simulink model "Solar_Panel_Tracking_Model"  (R2024b)
settings: Solver=VariableStepAuto  StartTime=0.0  StopTime=100  RelTol=1e-3
values from neighbouring files (symbols this model uses):
  J = 8.6    [Solar_Panel_Tracking_System.m]
  Kd = 8.6    [Solar_Panel_Tracking_System.m]
  Kf = 0.5    [Solar_Panel_Tracking_System.m]
  Kg = 1    [Solar_Panel_Tracking_System.m]
  Ki = 180    [Solar_Panel_Tracking_System.m]
  Kp = 240    [Solar_Panel_Tracking_System.m]
  Kt = 2    [Solar_Panel_Tracking_System.m]
  L = 1    [Solar_Panel_Tracking_System.m]
  R = 1.2    [Solar_Panel_Tracking_System.m]
libraries: slpidlib x1
settings Model: Creator=alexpadrpm  LastModifiedBy=alexpadrpm

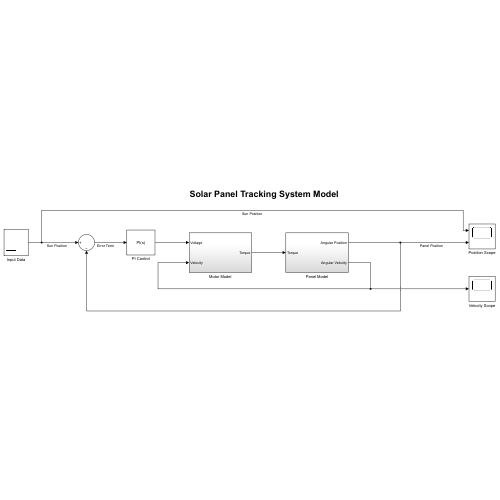
[thumbnail: Simulink's stored preview of the top-level diagram]
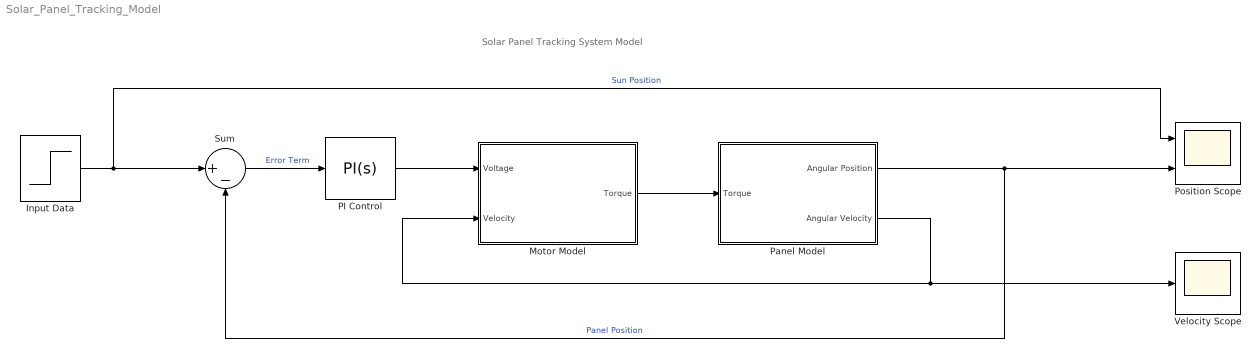
== system Solar_Panel_Tracking_Model ==
  note: Solar Panel Tracking System Model
  Input Data : Step  SampleTime=0
  Motor Model : Subsystem
  PI Control : slpidlib/PID Controller  Controller=PI  Form=Parallel  TimeDomain=Continuous-time  UseExternalTs=off  SampleTime=-1  IntegratorMethod=Forward Euler  FilterMethod=Forward Euler  ControllerParametersSource=internal  P=Kp  I=Ki  UseKiTs=off  D=0  UseExternalDerivativeSource=off  N=100  UseFilter=on  TunerSelectOption=Transfer Function Based (PID Tuner App)  InitialConditionSource=internal  InitialConditionForIntegrator=0  InitialConditionForFilter=0  DifferentiatorICPrevScaledInput=0  ExternalReset=none  TrackingMode=off  Kt=1  LimitOutput=off  SatLimitsSource=internal  UpperSaturationLimit=inf  LowerSaturationLimit=-inf  LinearizeAsGain=on  AntiWindupMode=none  Kb=1  LimitIntegrator=off  UpperIntegratorSaturationLimit=inf  LowerIntegratorSaturationLimit=-inf  POutMin=[]  POutMax=[]  IOutMin=[]  IOutMax=[]  DOutMin=[]  DOutMax=[]  NOutMin=[]  NOutMax=[]  SumOutMin=[]  SumOutMax=[]  SaturationOutMin=[]  SaturationOutMax=[]  PParamMin=[]  PParamMax=[]  IParamMin=[]  IParamMax=[]  DParamMin=[]  DParamMax=[]  NParamMin=[]  NParamMax=[]  KbParamMin=[]  KbParamMax=[]  KtParamMin=[]  KtParamMax=[]  KbOutMin=[]  KbOutMax=[]  KtOutMin=[]  KtOutMax=[]  IntegratorOutMin=[]  IntegratorOutMax=[]  FilterOutMin=[]  FilterOutMax=[]  SumI1OutMin=[]  SumI1OutMax=[]  SumI2OutMin=[]  SumI2OutMax=[]  SumI3OutMin=[]  SumI3OutMax=[]  SumI4OutMin=[]  SumI4OutMax=[]  SumDOutMin=[]  SumDOutMax=[]  DifferentiatorOutMin=[]  DifferentiatorOutMax=[]  FilterDiffOutCoefMin=[]  FilterDiffOutCoefMax=[]  ReciprocalOutMin=[]  ReciprocalOutMax=[]  SumDenOutMin=[]  SumDenOutMax=[]  SumNumOutMin=[]  SumNumOutMax=[]  DivideOutMin=[]  DivideOutMax=[]  UdiffTsProdOutMin=[]  UdiffTsProdOutMax=[]  NTsProdOutMin=[]  NTsProdOutMax=[]  UintegralTsProdOutMin=[]  UintegralTsProdOutMax=[]  UngainTsProdOutMin=[]  UngainTsProdOutMax=[]  ClampingZeroOutDataTypeStr=Inherit: Inherit via back propagation  ClampingZeroOutMin=[]  ClampingZeroOutMax=[]  FilterDenConstantOutDataTypeStr=Inherit: Inherit via back propagation  FilterDenConstantOutMin=[]  FilterDenConstantOutMax=[]  PCopyOutDataTypeStr=Inherit: Inherit via back propagation  PCopyOutMin=[]  PCopyOutMax=[]  NCopyOutDataTypeStr=Inherit: Inherit via back propagation  NCopyOutMin=[]  NCopyOutMax=[]  IntegratorContinuousStateAttributes=''  IntegratorStateMustResolveToSignalObject=off  IntegratorRTWStateStorageClass=Auto  FilterContinuousStateAttributes=''  FilterStateMustResolveToSignalObject=off  FilterRTWStateStorageClass=Auto  ParallelPVariant=InternalParameters  IdealPVariant=Disabled  IVariant=InternalParameters  DVariant=Disabled  IntegratorVariant=Continuous  SatVariant=Disabled  AWVariant=Passthrough  PCopyVariant=Disabled  TRVariant=Disabled  FdbkBlocksVariant=Forward  IdealPFdbkVariant=Disabled  SatFdbkVariant=Disabled  DerivativeFilterVariant=Disabled  NVariant=Disabled  NCopyVariant=Disabled_SignalSpec  FilterICVariant=Disabled  IntegratorICVariant=InternalICs  ExternalResetVariant=Disabled  TRSumVariant=Passthrough  SumFdbkVariant=Disabled  SumVariant=Sum_PI  TsampFilterVariant=InternalTs  TsampNgainVariant=Passthrough  TsampIntegralVariant=Disabled_SignalSpec  ExternalSaturationOutDataTypeStr=Inherit: Same as second input  DerivativeSourceVariant=Disabled  PreIntVariant=InternalPreInt
  Panel Model : Subsystem
  Position Scope : Scope  NumInputPorts=2
  Sum : Sum  Inputs=|+-
  Velocity Scope : Scope
  wires:
  Panel Model/2(Angular Velocity) -> Velocity Scope/1, Motor Model/2(Velocity)
  Motor Model/1(Torque) -> Panel Model/1(Torque)
  Input Data/1 -> Sum/1, Position Scope/1  "Sun Position"
  Panel Model/1(Angular Position) -> Sum/2, Position Scope/2  "Panel Position"
  Sum/1 -> PI Control/1  "Error Term"
  PI Control/1 -> Motor Model/1(Voltage)

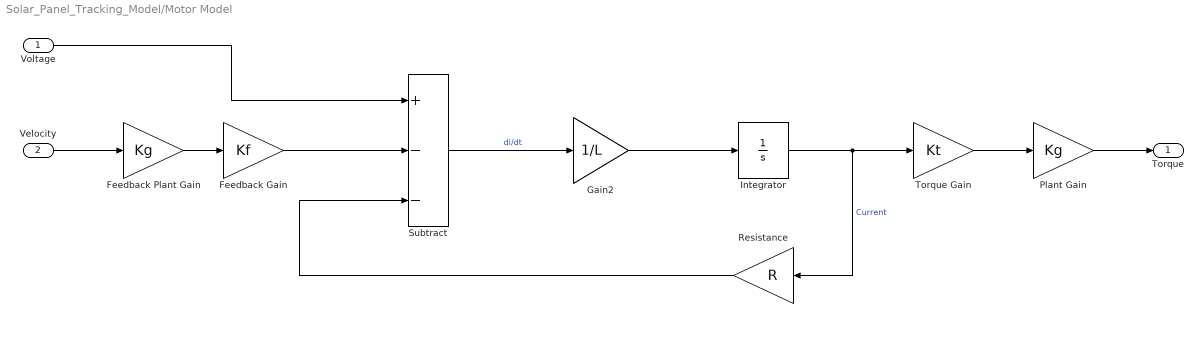
== system Solar_Panel_Tracking_Model/Motor Model ==
  Voltage : Inport
  Velocity : Inport  Port=2
  Feedback Gain : Gain  Gain=Kf
  Feedback Plant Gain : Gain  Gain=Kg
  Gain2 : Gain  Gain=1/L
  Integrator : Integrator
  Plant Gain : Gain  Gain=Kg
  Resistance : Gain  Gain=R
  Subtract : Sum  Inputs=+--
  Torque Gain : Gain  Gain=Kt
  Torque : Outport
  wires:
  Integrator/1 -> Resistance/1, Torque Gain/1  "Current"
  Subtract/1 -> Gain2/1  "di/dt"
  Voltage/1 -> Subtract/1
  Gain2/1 -> Integrator/1
  Torque Gain/1 -> Plant Gain/1
  Plant Gain/1 -> Torque/1
  Velocity/1 -> Feedback Plant Gain/1
  Feedback Plant Gain/1 -> Feedback Gain/1
  Feedback Gain/1 -> Subtract/2
  Resistance/1 -> Subtract/3

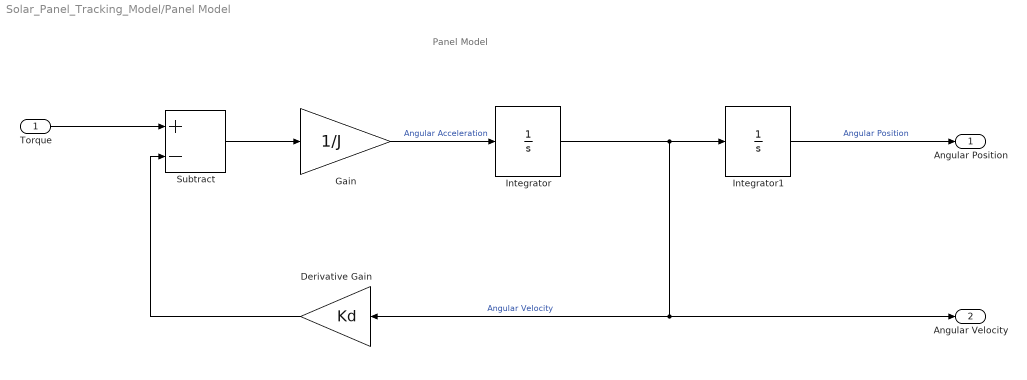
== system Solar_Panel_Tracking_Model/Panel Model ==
  note: Panel Model
  Torque : Inport
  Derivative Gain : Gain  Gain=Kd
  Gain : Gain  Gain=1/J
  Integrator : Integrator
  Integrator1 : Integrator
  Subtract : Sum  Inputs=+-
  Angular Position : Outport
  Angular Velocity : Outport  Port=2
  wires:
  Integrator/1 -> Angular Velocity/1, Derivative Gain/1, Integrator1/1  "Angular Velocity"
  Integrator1/1 -> Angular Position/1  "Angular Position"
  Torque/1 -> Subtract/1
  Subtract/1 -> Gain/1
  Gain/1 -> Integrator/1  "Angular Acceleration"
  Derivative Gain/1 -> Subtract/2
